simulink model "afe_dq_inv_psm"  (R2025a)
settings: Solver=ode1be  StartTime=0.0  StopTime=simlength  FixedStep=tc  MaxStep=tc
undefined symbols (not defined in the file): Adrso, Amplitude_U, Amplitude_V, Amplitude_W, b, Crso, CTRPIFF_CLIP_RELEASE, dead_time_AFE, dead_time_INV, deepNEGeta, deepNEGxi, deepPOSxi, emf_fb_p, emf_fb_p_ccaller_1, emf_fb_p_ccaller_2, emf_p, emf_p_ccaller_1, emf_p_ccaller_2, end_time_LVRT, fPWM_AFE, fPWM_INV, g0_500Hz, g1_500Hz, ibez, id_lim, Igrid_phase_normalization_factor, iq_lim, ixi_pos_ref_lim, Jm, kg, ki_afe, ki_i, ki_rc_grid, ki_vs, ki_w, kp_afe, kp_i, kp_rc_grid, kp_vs, kp_w, kw, Ld_norm, Ldrso, Lq_norm, Ls_norm, magnitude, motorc_m_scale, n1, n10, omega_bez, omega_grid_emulator_nom, omega_grid_nom, omega_m_bez, omega_m_sim, Phase_shift, pll_i1, pll_i1_ddsrt, pll_p, pll_p_ddsrt, pll_p_frt ... (+27)
libraries: fl_lib x114, nesl_utility x78, cstblocks x14, single_phase_transformer_lib x3, threephase_inductor_lib x2, simulink x2, flexshaft_lib x1, pmsm_uvw_with_harmonics_lib x1
(part 2 of 7)

== system afe_dq_inv_psm/grid/grid_emulator ==
  3ph_Dyg : Subsystem
  Controlled Voltage Source : fl_lib/Electrical/Electrical Sources/Controlled Voltage Source
  Controlled Voltage Source1 : fl_lib/Electrical/Electrical Sources/Controlled Voltage Source
  Controlled Voltage Source2 : fl_lib/Electrical/Electrical Sources/Controlled Voltage Source
  Electrical Reference : fl_lib/Electrical/Electrical Elements/Electrical Reference
  Simulink-PS Converter : nesl_utility/Simulink-PS Converter  PhysicalDomain=network_engine_domain  SubClassName=ps_input  LeftPortType=input  RightPortType=output  PseudoPeriodic=off  Frequencies=[]  NoiseDistribution=none  NoiseParameters=[]  Unit=V  AffineConversion=on  FilteringAndDerivatives=provide  SimscapeFilterOrder=1  InputFilterTimeConstant=0.001  UdotUserProvided=0
  Simulink-PS Converter1 : nesl_utility/Simulink-PS Converter  PhysicalDomain=network_engine_domain  SubClassName=ps_input  LeftPortType=input  RightPortType=output  PseudoPeriodic=off  Frequencies=[]  NoiseDistribution=none  NoiseParameters=[]  Unit=V  AffineConversion=on  FilteringAndDerivatives=provide  SimscapeFilterOrder=1  InputFilterTimeConstant=0.001  UdotUserProvided=0
  Simulink-PS Converter2 : nesl_utility/Simulink-PS Converter  PhysicalDomain=network_engine_domain  SubClassName=ps_input  LeftPortType=input  RightPortType=output  PseudoPeriodic=off  Frequencies=[]  NoiseDistribution=none  NoiseParameters=[]  Unit=V  AffineConversion=on  FilteringAndDerivatives=provide  SimscapeFilterOrder=1  InputFilterTimeConstant=0.001  UdotUserProvided=0
  Solver Configuration : nesl_utility/Solver Configuration  PhysicalDomain=network_engine_domain  SubClassName=solver  LeftPortType=input  RightPortType=generic  Tones=[]  Harmonics=[]  SimulateNoise=off  Profile=off  UseLocalSampling=off  EnableSwitchedLinearOptims=on  FrequencyDomain=off  UseCCode=off  RelTol=0.001  AbsTol=0.001  MinStep=1e-09  ToWorkspace=off  RevertToSquareIcSolve=off  NumHomotopyIterations=100  PhasorMode=off  PhasorModeNumHarmonics=1  ConsistencySolver=NEWTON_FTOL  IndexReductionMethod=DerivativeReplacement  DoDC=off  ResidualTolerance=1e-09  ConsistencyTolSource=GLOBAL  ConsistencyAbsTol=0.001  ConsistencyRelTol=0.001  ConsistencyTolFactor=0.001  UseLocalSolver=on  LocalSolverChoice=NE_BACKWARD_EULER_ADVANCER  ResolveIndetEquations=on  FunctionEvalNumThread=1  LocalSolverSampleTime=tc  DoFixedCost=on  MaxNonlinIter=3  MaxModeIter=2  ComputeImpulses=off  ImpulseIterations=2  LinearAlgebra=auto  LinearAlgebraNumThread=0  EquationFormulation=NE_TIME_EF  DelaysMemoryBudget=1024  AutomaticFiltering=on  FilteringTimeConstant=0.001  PartitionStorageMethod=AS_NEEDED  PartitionMemoryBudget=1024  PartitionMethod=ROBUST  MultibodyUseLocalSolver=off  MultibodyLocalSolverChoice=ODE1  MultibodyLocalSolverSampleTime=0.001
  grid_emulator : Subsystem
  threephase_vi_measures : Subsystem
  u1 : PMIOPort  Side=Right
  u2 : PMIOPort  Port=2  Side=Right
  u3 : PMIOPort  Port=3  Side=Right
  wires:
  grid_emulator/2(Vmb) -> Simulink-PS Converter1/1
  grid_emulator/3(Vmc) -> Simulink-PS Converter2/1
  grid_emulator/1(Vma) -> Simulink-PS Converter/1
  connections:
  Simulink-PS Converter/RConn1 -- Controlled Voltage Source/RConn1
  Simulink-PS Converter1/RConn1 -- Controlled Voltage Source1/RConn1
  Simulink-PS Converter2/RConn1 -- Controlled Voltage Source2/RConn1
  Electrical Reference/LConn1 -- Solver Configuration/RConn1 -- Controlled Voltage Source/RConn2 -- Controlled Voltage Source1/RConn2 -- Controlled Voltage Source2/RConn2
  3ph_Dyg/RConn1 -- u1/RConn1
  3ph_Dyg/RConn2 -- u2/RConn1
  3ph_Dyg/RConn3 -- u3/RConn1
  threephase_vi_measures/RConn1 -- 3ph_Dyg/LConn1
  threephase_vi_measures/RConn2 -- 3ph_Dyg/LConn2
  threephase_vi_measures/RConn3 -- 3ph_Dyg/LConn3
  Controlled Voltage Source/LConn1 -- threephase_vi_measures/LConn1
  Controlled Voltage Source1/LConn1 -- threephase_vi_measures/LConn2
  Controlled Voltage Source2/LConn1 -- threephase_vi_measures/LConn3

== system afe_dq_inv_psm/grid/instantaneus_power ==
  Vline : Inport
  Iline : Inport  Port=2
  Demux2 : Demux  Outputs=3
  Demux3 : Demux  Outputs=3
  Fcn1 : Fcn  Expr=u(1)/(sqrt(u(1)^2+u(2)^2))
  Gain2 : Gain  Gain=3/2
  Gain3 : Gain  Gain=3/2
  Mux1 : Mux  Inputs=2
  Product{,1..3} (4 alike) : Product  RndMeth=Zero
  Sum : Sum  Inputs=|++
  Sum1 : Sum  Inputs=|+-
  To Workspace1 : ToWorkspace  VariableName=va_line_rms_sim  SampleTime=ts_afe
      settings: MaxDataPoints=Ns_afe
  To Workspace2 : ToWorkspace  VariableName=vb_line_rms_sim  SampleTime=ts_afe
      settings: MaxDataPoints=Ns_afe
  To Workspace3 : ToWorkspace  VariableName=vc_line_rms_sim  SampleTime=ts_afe
      settings: MaxDataPoints=Ns_afe
  To Workspace4 : ToWorkspace  VariableName=ia_line_rms_sim  SampleTime=ts_afe
      settings: MaxDataPoints=Ns_afe
  To Workspace5 : ToWorkspace  VariableName=ib_line_rms_sim  SampleTime=ts_afe
      settings: MaxDataPoints=Ns_afe
  To Workspace6 : ToWorkspace  VariableName=ic_line_rms_sim  SampleTime=ts_afe
      settings: MaxDataPoints=Ns_afe
  To Workspace7 : ToWorkspace  VariableName=Pline_avg_sim  SampleTime=ts_afe
      settings: MaxDataPoints=Ns_afe
  To Workspace8 : ToWorkspace  VariableName=Qline_avg_sim  SampleTime=ts_afe
      settings: MaxDataPoints=Ns_afe
  abc2alphabeta : Subsystem
  "abc2alphabeta " : Subsystem
  mavg_11 : Subsystem
  mavg_12 : Subsystem
  rms : Subsystem
  rms1 : Subsystem
  rms2 : Subsystem
  rms3 : Subsystem
  rms4 : Subsystem
  rms5 : Subsystem
  tag scope: Pline_avg=global, Qline_avg=global, cos_phi_avg=global
  wires:
  Gain3/1 -> mavg_12/1(in), To Workspace8/1
  Gain2/1 -> mavg_11/1(in), To Workspace7/1
  Demux2/1 -> abc2alphabeta/1(a), rms/1(In1)
  Vline/1 -> Demux2/1
  Iline/1 -> Demux3/1
  abc2alphabeta/2(vline_beta) -> Product1/1, Product2/1
  "abc2alphabeta "/2(i_line_beta) -> Product3/1, Product1/2
  abc2alphabeta/1(vline_alpha) -> Product/1, Product3/2
  "abc2alphabeta "/1(i_line_alpha) -> Product2/2, Product/2
  Product/1 -> Sum/1
  Product1/1 -> Sum/2
  Product2/1 -> Sum1/1
  Product3/1 -> Sum1/2
  Sum1/1 -> Gain3/1
  Sum/1 -> Gain2/1
  Demux2/2 -> abc2alphabeta/2(b), rms1/1(In1)
  Demux2/3 -> abc2alphabeta/3(c), rms2/1(In1)
  Demux3/1 -> "abc2alphabeta "/1(a), rms3/1(In1)
  Demux3/2 -> "abc2alphabeta "/2(b), rms4/1(In1)
  Demux3/3 -> rms5/1(In1), "abc2alphabeta "/3(c)
  mavg_11/1(out) -> [Pline_avg]
  mavg_12/1(out) -> [Qline_avg]
  [Qline_avg] -> Mux1/2
  Mux1/1 -> Fcn1/1
  Fcn1/1 -> [cos_phi_avg]
  [Pline_avg] -> Mux1/1
  rms/1(Out1) -> To Workspace1/1
  rms2/1(Out1) -> To Workspace3/1
  rms1/1(Out1) -> To Workspace2/1
  rms5/1(Out1) -> To Workspace6/1
  rms4/1(Out1) -> To Workspace5/1
  rms3/1(Out1) -> To Workspace4/1

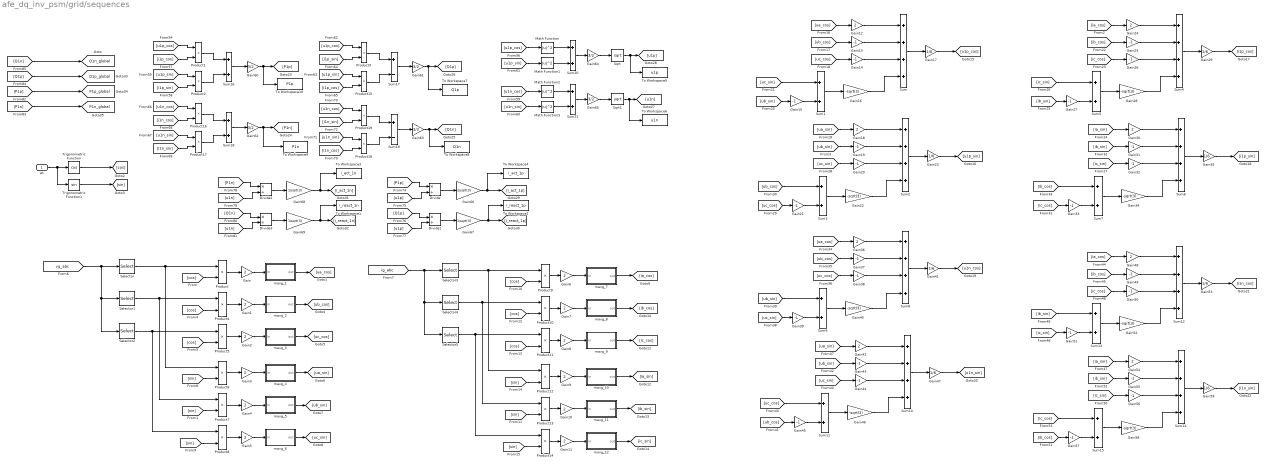
== system afe_dq_inv_psm/grid/sequences ==
  wt : Inport
  Divide{,1..3} (4 alike) : Product  Inputs=*/
  Gain{,1..12,18,24,30,36,42,48,54} (20 alike) : Gain  Gain=2
  Gain{13..15,19..21,25..27,31..33,37..39,43..45,49..51,55..57} (24 alike) : Gain  Gain=-1
  Gain{16,22,28,34,40,46,52,58} (8 alike) : Gain  Gain=-sqrt(3)
  Gain{17,23,29,35,41,47,53,59} (8 alike) : Gain  Gain=1/6
  Gain{60..65} (6 alike) : Gain  Gain=3/2
  Gain{66..69} (4 alike) : Gain  Gain=1/sqrt(3)
  Math Function{,1..3} (4 alike) : Math  Operator=magnitude^2  SignedPower=on
  Product{,1..19} (20 alike) : Product  RndMeth=Zero
  Selector : Selector  InputPortWidth=3  IndexOptions=Index vector (dialog)  Indices=1  OutputSizes=1
  Selector1 : Selector  InputPortWidth=3  IndexOptions=Index vector (dialog)  Indices=2  OutputSizes=1
  Selector2 : Selector  InputPortWidth=3  IndexOptions=Index vector (dialog)  Indices=3  OutputSizes=1
  Selector3 : Selector  InputPortWidth=3  IndexOptions=Index vector (dialog)  Indices=1  OutputSizes=1
  Selector4 : Selector  InputPortWidth=3  IndexOptions=Index vector (dialog)  Indices=2  OutputSizes=1
  Selector5 : Selector  InputPortWidth=3  IndexOptions=Index vector (dialog)  Indices=3  OutputSizes=1
  Sqrt : Sqrt
  Sqrt1 : Sqrt
  Sum{,2,4,6,8,10,12,14} (8 alike) : Sum  Inputs=++++
  Sum{1,3,5,7,9,11,13,15..16,18,20..21} (12 alike) : Sum
  Sum17 : Sum  Inputs=+-
  Sum19 : Sum  Inputs=+-
  To Workspace1 : ToWorkspace  VariableName=i_react_1n  SampleTime=ts_afe
      settings: MaxDataPoints=Ns_afe
  To Workspace10 : ToWorkspace  VariableName=P1p  SampleTime=ts_afe
      settings: MaxDataPoints=Ns_afe
  To Workspace2 : ToWorkspace  VariableName=i_react_1p  SampleTime=ts_afe
      settings: MaxDataPoints=Ns_afe
  To Workspace3 : ToWorkspace  VariableName=i_act_1n  SampleTime=ts_afe
      settings: MaxDataPoints=Ns_afe
  To Workspace4 : ToWorkspace  VariableName=i_act_1p  SampleTime=ts_afe
      settings: MaxDataPoints=Ns_afe
  To Workspace5 : ToWorkspace  VariableName=u1p  SampleTime=ts_afe
      settings: MaxDataPoints=Ns_afe
  To Workspace6 : ToWorkspace  VariableName=u1n  SampleTime=ts_afe
      settings: MaxDataPoints=Ns_afe
  To Workspace7 : ToWorkspace  VariableName=Q1p  SampleTime=ts_afe
      settings: MaxDataPoints=Ns_afe
  To Workspace8 : ToWorkspace  VariableName=Q1n  SampleTime=ts_afe
      settings: MaxDataPoints=Ns_afe
  To Workspace9 : ToWorkspace  VariableName=P1n  SampleTime=ts_afe
      settings: MaxDataPoints=Ns_afe
  Trigonometric Function : Trigonometry  Operator=cos
  Trigonometric Function1 : Trigonometry
  mavg_1 : Subsystem
  mavg_10 : Subsystem
  mavg_11 : Subsystem
  mavg_12 : Subsystem
  mavg_2 : Subsystem
  mavg_3 : Subsystem
  mavg_4 : Subsystem
  mavg_5 : Subsystem
  mavg_6 : Subsystem
  mavg_7 : Subsystem
  mavg_8 : Subsystem
  mavg_9 : Subsystem
  tag scope: P1n_global=global, P1p_global=global, Q1n_global=global, Q1p_global=global
  wires:
  [vg_abc] -> Selector2/1, Selector1/1, Selector/1
  Trigonometric Function1/1 -> [sin]
  Trigonometric Function/1 -> [cos]
  wt/1 -> Trigonometric Function/1, Trigonometric Function1/1
  [cos] -> Product/2
  Product/1 -> Gain/1
  [cos] -> Product4/2
  Product4/1 -> Gain1/1
  [cos] -> Product5/2
  Product5/1 -> Gain2/1
  [sin] -> Product6/2
  Selector/1 -> Product6/1, Product/1
  Product6/1 -> Gain3/1
  [sin] -> Product7/2
  Selector1/1 -> Product7/1, Product4/1
  Product7/1 -> Gain4/1
  [sin] -> Product8/2
  Selector2/1 -> Product8/1, Product5/1
  Product8/1 -> Gain5/1
  [ig_abc] -> Selector3/1, Selector4/1, Selector5/1
  [cos] -> Product9/2
  Product9/1 -> Gain6/1
  [cos] -> Product10/2
  Product10/1 -> Gain7/1
  [cos] -> Product11/2
  Product11/1 -> Gain8/1
  [sin] -> Product12/2
  Selector3/1 -> Product9/1, Product12/1
  Product12/1 -> Gain9/1
  [sin] -> Product13/2
  Selector4/1 -> Product10/1, Product13/1
  Product13/1 -> Gain10/1
  [sin] -> Product14/2
  Selector5/1 -> Product11/1, Product14/1
  Product14/1 -> Gain11/1
  Gain/1 -> mavg_1/1(in)
  mavg_1/1(out) -> [ua_cos]
  Gain1/1 -> mavg_2/1(in)
  Gain2/1 -> mavg_3/1(in)
  Gain3/1 -> mavg_4/1(in)
  Gain4/1 -> mavg_5/1(in)
  Gain5/1 -> mavg_6/1(in)
  Gain6/1 -> mavg_7/1(in)
  Gain7/1 -> mavg_8/1(in)
  Gain8/1 -> mavg_9/1(in)
  Gain9/1 -> mavg_10/1(in)
  Gain10/1 -> mavg_11/1(in)
  Gain11/1 -> mavg_12/1(in)
  [ua_cos] -> Gain12/1
  [ub_cos] -> Gain13/1
  [uc_cos] -> Gain14/1
  [uc_sin] -> Sum1/1
  Gain15/1 -> Sum1/2
  [ub_sin] -> Gain15/1
  Sum1/1 -> Gain16/1
  Gain16/1 -> Sum/4
  Gain14/1 -> Sum/3
  Gain13/1 -> Sum/2
  Gain12/1 -> Sum/1
  Sum/1 -> Gain17/1
  Gain17/1 -> [u1p_cos]
  [ua_sin] -> Gain18/1
  [ub_sin] -> Gain19/1
  [uc_sin] -> Gain20/1
  [ub_cos] -> Sum3/1
  Gain21/1 -> Sum3/2
  [uc_cos] -> Gain21/1
  Sum3/1 -> Gain22/1
  Gain22/1 -> Sum2/4
  Gain20/1 -> Sum2/3
  Gain19/1 -> Sum2/2
  Gain18/1 -> Sum2/1
  Sum2/1 -> Gain23/1
  Gain23/1 -> [u1p_sin]
  [ia_cos] -> Gain24/1
  [ib_cos] -> Gain25/1
  [ic_cos] -> Gain26/1
  [ic_sin] -> Sum5/1
  Gain27/1 -> Sum5/2
  [ib_sin] -> Gain27/1
  Sum5/1 -> Gain28/1
  Gain28/1 -> Sum4/4
  Gain26/1 -> Sum4/3
  Gain25/1 -> Sum4/2
  Gain24/1 -> Sum4/1
  Sum4/1 -> Gain29/1
  Gain29/1 -> [i1p_cos]
  [ia_sin] -> Gain30/1
  [ib_sin] -> Gain31/1
  [ic_sin] -> Gain32/1
  [ib_cos] -> Sum7/1
  Gain33/1 -> Sum7/2
  [ic_cos] -> Gain33/1
  Sum7/1 -> Gain34/1
  Gain34/1 -> Sum6/4
  Gain32/1 -> Sum6/3
  Gain31/1 -> Sum6/2
  Gain30/1 -> Sum6/1
  Sum6/1 -> Gain35/1
  Gain35/1 -> [i1p_sin]
  [ua_cos] -> Gain36/1
  [ub_cos] -> Gain37/1
  [uc_cos] -> Gain38/1
  [ub_sin] -> Sum9/1
  Gain39/1 -> Sum9/2
  [uc_sin] -> Gain39/1
  Sum9/1 -> Gain40/1
  Gain40/1 -> Sum8/4
  Gain38/1 -> Sum8/3
  Gain37/1 -> Sum8/2
  Gain36/1 -> Sum8/1
  Sum8/1 -> Gain41/1
  Gain41/1 -> [u1n_cos]
  [ua_sin] -> Gain42/1
  [ub_sin] -> Gain43/1
  [uc_sin] -> Gain44/1
  [uc_cos] -> Sum11/1
  Gain45/1 -> Sum11/2
  [ub_cos] -> Gain45/1
  Sum11/1 -> Gain46/1
  Gain46/1 -> Sum10/4
  Gain44/1 -> Sum10/3
  Gain43/1 -> Sum10/2
  Gain42/1 -> Sum10/1
  Sum10/1 -> Gain47/1
  Gain47/1 -> [u1n_sin]
  [ia_cos] -> Gain48/1
  [ib_cos] -> Gain49/1
  [ic_cos] -> Gain50/1
  [ib_sin] -> Sum13/1
  Gain51/1 -> Sum13/2
  [ic_sin] -> Gain51/1
  Sum13/1 -> Gain52/1
  Gain52/1 -> Sum12/4
  Gain50/1 -> Sum12/3
  Gain49/1 -> Sum12/2
  Gain48/1 -> Sum12/1
  Sum12/1 -> Gain53/1
  Gain53/1 -> [i1n_cos]
  [ia_sin] -> Gain54/1
  [ib_sin] -> Gain55/1
  [ic_sin] -> Gain56/1
  [ic_cos] -> Sum15/1
  Gain57/1 -> Sum15/2
  [ib_cos] -> Gain57/1
  Sum15/1 -> Gain58/1
  Gain58/1 -> Sum14/4
  Gain56/1 -> Sum14/3
  Gain55/1 -> Sum14/2
  Gain54/1 -> Sum14/1
  Sum14/1 -> Gain59/1
  Gain59/1 -> [i1n_sin]
  Sum16/1 -> Gain60/1
  Product1/1 -> Sum16/1
  Product2/1 -> Sum16/2
  Gain60/1 -> To Workspace10/1, [P1p]
  [u1p_cos] -> Product1/1
  [i1p_cos] -> Product1/2
  [u1p_sin] -> Product2/1
  [i1p_sin] -> Product2/2
  Sum17/1 -> Gain61/1
  Product3/1 -> Sum17/1
  Product15/1 -> Sum17/2
  Gain61/1 -> To Workspace7/1, [Q1p]
  [u1p_cos] -> Product3/1
  [i1p_sin] -> Product3/2
  [u1p_sin] -> Product15/1
  [i1p_cos] -> Product15/2
  Sum18/1 -> Gain62/1
  Product16/1 -> Sum18/1
  Product17/1 -> Sum18/2
  Gain62/1 -> To Workspace9/1, [P1n]
  [u1n_cos] -> Product16/1
  [i1n_cos] -> Product16/2
  [u1n_sin] -> Product17/1
  [i1n_sin] -> Product17/2
  Sum19/1 -> Gain63/1
  Product19/1 -> Sum19/1
  Product18/1 -> Sum19/2
  Gain63/1 -> To Workspace8/1, [Q1n]
  [u1n_cos] -> Product19/1
  [i1n_sin] -> Product19/2
  [u1n_sin] -> Product18/1
  [i1n_cos] -> Product18/2
  [u1p_cos] -> Math Function/1
  [u1p_sin] -> Math Function1/1
  Math Function/1 -> Sum20/1
  Math Function1/1 -> Sum20/2
  Sum20/1 -> Gain64/1
  Gain64/1 -> Sqrt/1
  Sqrt/1 -> To Workspace5/1, [u1p]
  [u1n_cos] -> Math Function2/1
  [u1n_sin] -> Math Function3/1
  Math Function2/1 -> Sum21/1
  Math Function3/1 -> Sum21/2
  Sum21/1 -> Gain65/1
  Gain65/1 -> Sqrt1/1
  Sqrt1/1 -> To Workspace6/1, [u1n]
  [P1p] -> Divide/1
  [u1p] -> Divide/2
  Divide/1 -> Gain66/1
  Gain66/1 -> To Workspace4/1, [i_act_1p]
  [Q1p] -> Divide1/1
  [u1p] -> Divide1/2
  Divide1/1 -> Gain67/1
  Gain67/1 -> To Workspace2/1, [i_react_1p]
  [P1n] -> Divide2/1
  [u1n] -> Divide2/2
  Divide2/1 -> Gain68/1
  Gain68/1 -> To Workspace3/1, [i_act_1n]
  [Q1n] -> Divide3/1
  [u1n] -> Divide3/2
  Divide3/1 -> Gain69/1
  Gain69/1 -> To Workspace1/1, [i_react_1n]
  mavg_2/1(out) -> [ub_cos]
  mavg_3/1(out) -> [uc_cos]
  mavg_4/1(out) -> [ua_sin]
  mavg_5/1(out) -> [ub_sin]
  mavg_6/1(out) -> [uc_sin]
  mavg_7/1(out) -> [ia_cos]
  mavg_8/1(out) -> [ib_cos]
  mavg_9/1(out) -> [ic_cos]
  mavg_10/1(out) -> [ia_sin]
  mavg_11/1(out) -> [ib_sin]
  mavg_12/1(out) -> [ic_sin]
  [Q1n] -> [Q1n_global]
  [Q1p] -> [Q1p_global]
  [P1p] -> [P1p_global]
  [P1n] -> [P1n_global]

== system afe_dq_inv_psm/grid/threephase_vi_measures ==
  Bus Creator : BusCreator  Inputs=6
  Current Sensor : fl_lib/Electrical/Electrical Sensors/Current Sensor
  Current Sensor1 : fl_lib/Electrical/Electrical Sensors/Current Sensor
  Current Sensor2 : fl_lib/Electrical/Electrical Sensors/Current Sensor
  Electrical Reference1 : fl_lib/Electrical/Electrical Elements/Electrical Reference
  Selector : Selector  InputPortWidth=6  IndexOptions=Index vector (dialog)  Indices=[1 2 3]  OutputSizes=1
  Selector1 : Selector  InputPortWidth=6  IndexOptions=Index vector (dialog)  Indices=[4 5 6]  OutputSizes=1
  Voltage Sensor : fl_lib/Electrical/Electrical Sensors/Voltage Sensor
  Voltage Sensor1 : fl_lib/Electrical/Electrical Sensors/Voltage Sensor
  Voltage Sensor2 : fl_lib/Electrical/Electrical Sensors/Voltage Sensor
  ia_grid : nesl_utility/PS-Simulink Converter  PhysicalDomain=network_engine_domain  SubClassName=ps_output  LeftPortType=input  RightPortType=output  PseudoPeriodic=off  Frequencies=[]  VectorFormat=1-D array  Unit=A  AffineConversion=off
  ib_grid : nesl_utility/PS-Simulink Converter  PhysicalDomain=network_engine_domain  SubClassName=ps_output  LeftPortType=input  RightPortType=output  PseudoPeriodic=off  Frequencies=[]  VectorFormat=1-D array  Unit=A  AffineConversion=off
  ic_grid : nesl_utility/PS-Simulink Converter  PhysicalDomain=network_engine_domain  SubClassName=ps_output  LeftPortType=input  RightPortType=output  PseudoPeriodic=off  Frequencies=[]  VectorFormat=1-D array  Unit=A  AffineConversion=off
  ig_abc/ug_abc : Scope  NumInputPorts=2
      settings: SampleTime=tc  ActiveDisplayYMinimum=-728.04682585664023  ActiveDisplayYMaximum=740.95420771528393  DataLoggingVariableName=ScopeData2
  power-meter : Scope  NumInputPorts=2
      settings: SampleTime=tc  ActiveDisplayYMinimum=-388201.13873747073  ActiveDisplayYMaximum=116083.0892842215  DataLoggingVariableName=ScopeData3
  ua_grid : nesl_utility/PS-Simulink Converter  PhysicalDomain=network_engine_domain  SubClassName=ps_output  LeftPortType=input  RightPortType=output  PseudoPeriodic=off  Frequencies=[]  VectorFormat=1-D array  Unit=V  AffineConversion=off
  ub_grid : nesl_utility/PS-Simulink Converter  PhysicalDomain=network_engine_domain  SubClassName=ps_output  LeftPortType=input  RightPortType=output  PseudoPeriodic=off  Frequencies=[]  VectorFormat=1-D array  Unit=V  AffineConversion=off
  uc_grid : nesl_utility/PS-Simulink Converter  PhysicalDomain=network_engine_domain  SubClassName=ps_output  LeftPortType=input  RightPortType=output  PseudoPeriodic=off  Frequencies=[]  VectorFormat=1-D array  Unit=V  AffineConversion=off
  Ua : PMIOPort  Side=Left
  ua : PMIOPort  Port=2  Side=Right
  Ub : PMIOPort  Port=3  Side=Left
  ub : PMIOPort  Port=4  Side=Right
  Uc : PMIOPort  Port=5  Side=Left
  uc : PMIOPort  Port=6  Side=Right
  tag scope: ig_abc=global, vg_abc=global
  wires:
  Bus Creator/1 -> Selector1/1, Selector/1  "vi_data"
  Selector/1 -> [vg_abc]
  ib_grid/1 -> Bus Creator/5  "ib"
  ia_grid/1 -> Bus Creator/4  "ia"
  ic_grid/1 -> Bus Creator/6  "ic"
  ua_grid/1 -> Bus Creator/1  "ua"
  ub_grid/1 -> Bus Creator/2  "ub"
  uc_grid/1 -> Bus Creator/3  "uc"
  Selector1/1 -> [ig_abc]
  [vg_abc] -> ig_abc/ug_abc/2
  [ig_abc] -> ig_abc/ug_abc/1
  [Pline_avg] -> power-meter/1
  [Qline_avg] -> power-meter/2
  connections:
  Current Sensor1/LConn1 -- Ub/RConn1 -- Voltage Sensor1/LConn1
  Electrical Reference1/LConn1 -- Voltage Sensor/RConn2 -- Voltage Sensor2/RConn2 -- Voltage Sensor1/RConn2
  Voltage Sensor/RConn1 -- ua_grid/LConn1
  Current Sensor/RConn2 -- ua/RConn1
  Voltage Sensor1/RConn1 -- ub_grid/LConn1
  Voltage Sensor2/LConn1 -- Current Sensor2/LConn1 -- Uc/RConn1
  Current Sensor/LConn1 -- Ua/RConn1 -- Voltage Sensor/LConn1
  Current Sensor1/RConn2 -- ub/RConn1
  Voltage Sensor2/RConn1 -- uc_grid/LConn1
  ib_grid/LConn1 -- Current Sensor1/RConn1
  ia_grid/LConn1 -- Current Sensor/RConn1
  ic_grid/LConn1 -- Current Sensor2/RConn1
  Current Sensor2/RConn2 -- uc/RConn1

== system afe_dq_inv_psm/motor_load_setting/flex-shaft ==
  flexible shaft : flexshaft_lib/flexible shaft  b1=1 N*m*s/rad  J1=1 kg*m^2  b2=1 N*m*s/rad  J2=1 kg*m^2  b_theta=1 N*m*s/rad  k_theta=1e4 N*m/rad  w_1_specify=off  w_1_priority=None  w_1=0 rad/s  w_1_nominal_specify=off  w_1_nominal_value=1  w_1_nominal_unit=rad/s  w_2_specify=off  w_2_priority=None  w_2=0 rad/s  w_2_nominal_specify=off  w_2_nominal_value=1  w_2_nominal_unit=rad/s  t_1_specify=off  t_1_priority=None  t_1=0 N*m  t_1_nominal_specify=off  t_1_nominal_value=1  t_1_nominal_unit=N*m  t_2_specify=off  t_2_priority=None  t_2=0 N*m  t_2_nominal_specify=off  t_2_nominal_value=1  t_2_nominal_unit=N*m  t_theta_specify=off  t_theta_priority=None  t_theta=0 N*m  t_theta_nominal_specify=off  t_theta_nominal_value=1  t_theta_nominal_unit=N*m
      settings: InternalSimscapePortConfiguration="{\"Bottom\":[],\"Left\":[{\"id\":\"S1\",\"label\":\"S1\",\"type\":\"foundation.mechanical.rotational.rotational\"}],\"Right\":[{\"id\":\"S2\",\"label\":\"S2\",\"type\":\"foundation.mechanical.rotational.rotational\"}],\"Top\":[]}"
  s2 : PMIOPort  Side=Right
  s1 : PMIOPort  Port=2  Side=Left
  connections:
  flexible shaft/RConn1 -- s2/RConn1
  flexible shaft/LConn1 -- s1/RConn1

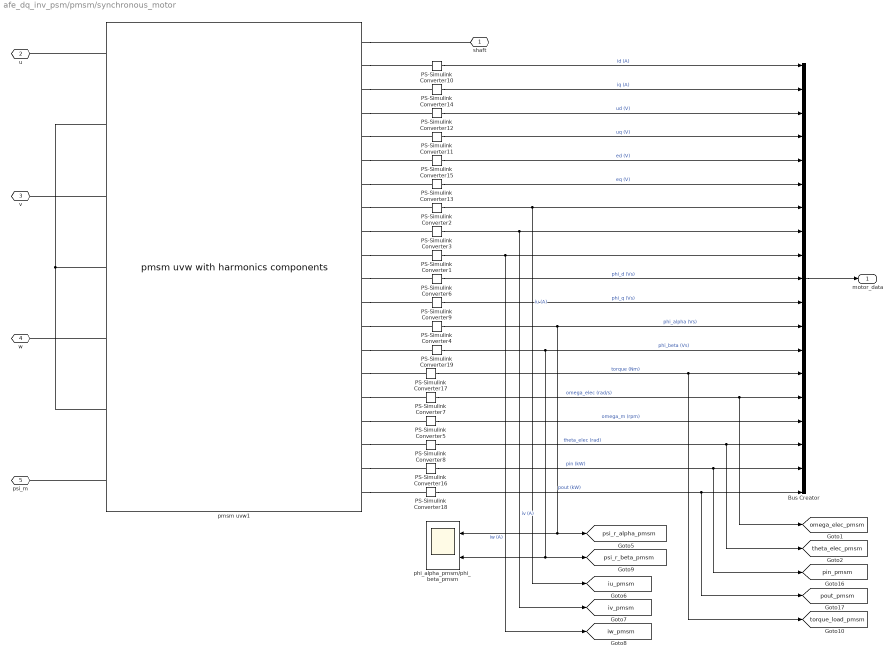
== system afe_dq_inv_psm/pmsm/synchronous_motor ==
  Bus Creator : BusCreator  Inputs=19
  PS-Simulink Converter{1..3,10,14} (5 alike) : nesl_utility/PS-Simulink Converter  PhysicalDomain=network_engine_domain  SubClassName=ps_output  LeftPortType=input  RightPortType=output  PseudoPeriodic=off  Frequencies=[]  VectorFormat=1-D array  Unit=A  AffineConversion=off
  PS-Simulink Converter{11..13,15} (4 alike) : nesl_utility/PS-Simulink Converter  PhysicalDomain=network_engine_domain  SubClassName=ps_output  LeftPortType=input  RightPortType=output  PseudoPeriodic=off  Frequencies=[]  VectorFormat=1-D array  Unit=V  AffineConversion=off
  PS-Simulink Converter16 : nesl_utility/PS-Simulink Converter  PhysicalDomain=network_engine_domain  SubClassName=ps_output  LeftPortType=input  RightPortType=output  PseudoPeriodic=off  Frequencies=[]  VectorFormat=1-D array  Unit=kW  AffineConversion=off
  PS-Simulink Converter17 : nesl_utility/PS-Simulink Converter  PhysicalDomain=network_engine_domain  SubClassName=ps_output  LeftPortType=input  RightPortType=output  PseudoPeriodic=off  Frequencies=[]  VectorFormat=1-D array  Unit=N*m  AffineConversion=off
  PS-Simulink Converter18 : nesl_utility/PS-Simulink Converter  PhysicalDomain=network_engine_domain  SubClassName=ps_output  LeftPortType=input  RightPortType=output  PseudoPeriodic=off  Frequencies=[]  VectorFormat=1-D array  Unit=kW  AffineConversion=off
  PS-Simulink Converter{4,6,9,19} (4 alike) : nesl_utility/PS-Simulink Converter  PhysicalDomain=network_engine_domain  SubClassName=ps_output  LeftPortType=input  RightPortType=output  PseudoPeriodic=off  Frequencies=[]  VectorFormat=1-D array  Unit=V*s  AffineConversion=off
  PS-Simulink Converter5 : nesl_utility/PS-Simulink Converter  PhysicalDomain=network_engine_domain  SubClassName=ps_output  LeftPortType=input  RightPortType=output  PseudoPeriodic=off  Frequencies=[]  VectorFormat=1-D array  Unit=rpm  AffineConversion=off
  PS-Simulink Converter7 : nesl_utility/PS-Simulink Converter  PhysicalDomain=network_engine_domain  SubClassName=ps_output  LeftPortType=input  RightPortType=output  PseudoPeriodic=off  Frequencies=[]  VectorFormat=1-D array  Unit=rad/s  AffineConversion=off
  PS-Simulink Converter8 : nesl_utility/PS-Simulink Converter  PhysicalDomain=network_engine_domain  SubClassName=ps_output  LeftPortType=input  RightPortType=output  PseudoPeriodic=off  Frequencies=[]  VectorFormat=1-D array  Unit=rad  AffineConversion=off
  phi_alpha_pmsm/phi_beta_pmsm : Scope  NumInputPorts=2
      settings: SampleTime=tc  ActiveDisplayYMinimum=-4.80078  ActiveDisplayYMaximum=4.80088  DataLoggingVariableName=ScopeData2
  pmsm uvw1 : pmsm_uvw_with_harmonics_lib/pmsm uvw with harmonics components  number_poles=number_poles  psi_m_p=psi_m V*s  Lmu=Lmu H  La=La H  Lb=Lb H  Rs=Rs Ohm  J=Jm kg*m^2  b=b N*m*s/rad  b_square=0 %b_square N*m*s^2/rad^2  h5=4 percent  h7=1 percent  angle_error=0 rad  omega_specify=off  omega_priority=None  omega=0 rad/s  omega_nominal_specify=off  omega_nominal_unit=rad/s  omega_nominal_value=1  theta_specify=off  theta_priority=High  theta=0 rad  theta_nominal_specify=off  theta_nominal_unit=rad  theta_nominal_value=1  iu_specify=off  iu_priority=None  iu=0 A  iu_nominal_specify=off  iu_nominal_unit=A  iu_nominal_value=1  iv_specify=off  iv_priority=None  iv=0 A  iv_nominal_specify=off  iv_nominal_unit=A  iv_nominal_value=1  iw_specify=off  iw_priority=None  iw=0 A  iw_nominal_specify=off  iw_nominal_unit=A  iw_nominal_value=1  id_specify=off  id_priority=None  id=0 A  id_nominal_specify=off  id_nominal_unit=A  id_nominal_value=1  iq_specify=off  iq_priority=None  iq=0 A  iq_nominal_specify=off  iq_nominal_unit=A  iq_nominal_value=1  uv_specify=off  uv_priority=None  uv=0 V  uv_nominal_specify=off  uv_nominal_unit=V  uv_nominal_value=1  uu_specify=off  uu_priority=None  uu=0 V  uu_nominal_specify=off  uu_nominal_unit=V  uu_nominal_value=1  uw_specify=off  uw_priority=None  uw=0 V  uw_nominal_specify=off  uw_nominal_unit=V  uw_nominal_value=1  ud_specify=off  ud_priority=None  ud=0 V  ud_nominal_specify=off  ud_nominal_unit=V  ud_nominal_value=1  uq_specify=off  uq_priority=None  uq=0 V  uq_nominal_specify=off  uq_nominal_unit=V  uq_nominal_value=1  psi_r_u_specify=on  psi_r_u_priority=High  psi_r_u=psi_m V*s  psi_r_u_nominal_specify=off  psi_r_u_nominal_unit=V*s  psi_r_u_nominal_value=1  psi_r_v_specify=on  psi_r_v_priority=High  psi_r_v=-psi_m/2 V*s  psi_r_v_nominal_specify=off  psi_r_v_nominal_unit=V*s  psi_r_v_nominal_value=1  psi_r_w_specify=on  psi_r_w_priority=High  psi_r_w=-psi_m/2 V*s  psi_r_w_nominal_specify=off  psi_r_w_nominal_unit=V*s  psi_r_w_nominal_value=1  psi_s_d_specify=off  psi_s_d_priority=None  psi_s_d=0.0 V*s  psi_s_d_nominal_specify=off  psi_s_d_nominal_unit=V*s  psi_s_d_nominal_value=1  psi_s_q_specify=off  psi_s_q_priority=None  psi_s_q=0.0 V*s  psi_s_q_nominal_specify=off  psi_s_q_nominal_unit=V*s  psi_s_q_nominal_value=1  psi_r_d_specify=off  psi_r_d_priority=High  psi_r_d=phi_m V*s  psi_r_d_nominal_specify=off  psi_r_d_nominal_unit=V*s  psi_r_d_nominal_value=1  psi_r_q_specify=off  psi_r_q_priority=High  psi_r_q=0.0 V*s  psi_r_q_nominal_specify=off  psi_r_q_nominal_unit=V*s  psi_r_q_nominal_value=1  psi_r_alpha_specify=off  psi_r_alpha_priority=High  psi_r_alpha=psi_m V*s  psi_r_alpha_nominal_specify=off  psi_r_alpha_nominal_unit=V*s  psi_r_alpha_nominal_value=1  psi_r_beta_specify=off  psi_r_beta_priority=High  psi_r_beta=0 V*s  psi_r_beta_nominal_specify=off  psi_r_beta_nominal_unit=V*s  psi_r_beta_nominal_value=1  psi_s_alpha_specify=off  psi_s_alpha_priority=None  psi_s_alpha=0.0 V*s  psi_s_alpha_nominal_specify=off  psi_s_alpha_nominal_unit=V*s  psi_s_alpha_nominal_value=1  psi_s_beta_specify=off  psi_s_beta_priority=None  psi_s_beta=0.0 V*s  psi_s_beta_nominal_specify=off  psi_s_beta_nominal_unit=V*s  psi_s_beta_nominal_value=1  tau_l_specify=off  tau_l_priority=None  tau_l=0 N*m  tau_l_nominal_specify=off  tau_l_nominal_unit=N*m  tau_l_nominal_value=1  tau_m_specify=off  tau_m_priority=None  tau_m=0 N*m  tau_m_nominal_specify=off  tau_m_nominal_unit=N*m  tau_m_nominal_value=1
      settings: InternalSimscapePortConfiguration="{\"Bottom\":[],\"Left\":[{\"id\":\"uu_p\",\"label\":\"_uu+_\",\"type\":\"foundation.electrical.electrical\"},{\"id\":\"uu_n\",\"label\":\"_uu-_\",\"type\":\"foundation.electrical.electrical\"},{\"id\":\"uv_p\",\"label\":\"_uv+_\",\"type\":\"foundation.electrical.electrical\"},{\"id\":\"uv_n\",\"label\":\"_uv-_\",\"type\":\"foundation.electrical.electrical\"},{\"id\":\"uw_p\",\"label\":\"_uw+_\",\"type\":\"foundation.electrical.electrical\"},{\"id\":\"uw_n\",\"label\":\"_uw-_\",\"type\":\"foundation.electrical.electrical\"},{\"id\":\"psi_m\",\"label\":\"_psi_m_\",\"type\":\"input\"}],\"Right\":[{\"id\":\"S\",\"label\":\"_S_\",\"type\":\"foundation.mechanical.rotational.rotational\"},{\"id\":\"id_out\",\"label\":\"_id_\",\"type\":\"output\"},{\"id\":\"iq_out\",\"label\":\"_iq_\",\"type\":\"output\"},{\"id\":\"ud_out\",\"label\":\"_ud_\",\"type\":\"output\"},{\"id\":\"uq_out\",\"label\":\"_uq_\",\"type\":\"output\"},{\"id\":\"ed_out\",\"label\":\"_ed_\",\"type\":\"output\"},{\"id\":\"eq_out\",\"label\":\"_eq_\",\"type\":\"output\"},{\"id\":\"iu_out\",\"label\":\"_iu_\",\"type\":\"output\"},{\"id\":\"iv_out\",\"label\":\"_iv_\",\"type\":\"output\"},{\"id\":\"iw_out\",\"label\":\"_iw_\",\"type\":\"output\"},{\"id\":\"psi_r_d_out\",\"label\":\"_psi_r_d_\",\"type\":\"output\"},{\"id\":\"psi_r_q_out\",\"label\":\"_psi_r_q\",\"type\":\"output\"},{\"id\":\"psi_r_alpha_out\",\"label\":\"_psi_r_alpha_\",\"type\":\"output\"},{\"id\":\"psi_r_beta_out\",\"label\":\"_psi_r_beta\",\"type\":\"output\"},{\"id\":\"tau_out\",\"label\":\"_torque_\",\"type\":\"output\"},{\"id\":\"omega_out\",\"label\":\"_omega_elec_\",\"type\":\"output\"},{\"id\":\"omega_m_out\",\"label\":\"_omega_m_\",\"type\":\"output\"},{\"id\":\"theta_out\",\"label\":\"_theta_elec_\",\"type\":\"output\"},{\"id\":\"pin_out\",\"label\":\"_pin_\",\"type\":\"output\"},{\"id\":\"pout_out\",\"label\":\"_pout_\",\"type\":\"output\"}],\"Top\":[]}"
  shaft : PMIOPort  Side=Right
  u : PMIOPort  Port=2  Side=Left
  v : PMIOPort  Port=3  Side=Left
  w : PMIOPort  Port=4  Side=Left
  psi_m : PMIOPort  Port=5  Side=Left
  motor_data : Outport
  tag scope: iu_pmsm=global, iv_pmsm=global, iw_pmsm=global, omega_elec_pmsm=global, pin_pmsm=global, pout_pmsm=global, psi_r_alpha_pmsm=global, psi_r_beta_pmsm=global, theta_elec_pmsm=global, torque_load_pmsm=global
  wires:
  PS-Simulink Converter10/1 -> Bus Creator/1  "id (A)"
  PS-Simulink Converter14/1 -> Bus Creator/2  "iq (A)"
  PS-Simulink Converter12/1 -> Bus Creator/3  "ud (V)"
  PS-Simulink Converter11/1 -> Bus Creator/4  "uq (V)"
  PS-Simulink Converter15/1 -> Bus Creator/5  "ed (V)"
  PS-Simulink Converter13/1 -> Bus Creator/6  "eq (V)"
  PS-Simulink Converter2/1 -> Bus Creator/7, [iu_pmsm]  "iu (A)"
  PS-Simulink Converter3/1 -> Bus Creator/8, [iv_pmsm]  "iv (A)"
  PS-Simulink Converter1/1 -> Bus Creator/9, [iw_pmsm]  "iw (A)"
  PS-Simulink Converter6/1 -> Bus Creator/10  "phi_d (Vs)"
  PS-Simulink Converter9/1 -> Bus Creator/11  "phi_q (Vs)"
  Bus Creator/1 -> motor_data/1
  PS-Simulink Converter18/1 -> Bus Creator/19, [pout_pmsm]  "pout (kW)"
  PS-Simulink Converter16/1 -> Bus Creator/18, [pin_pmsm]  "pin (kW)"
  PS-Simulink Converter8/1 -> Bus Creator/17, [theta_elec_pmsm]  "theta_elec (rad)"
  PS-Simulink Converter5/1 -> Bus Creator/16  "omega_m (rpm)"
  PS-Simulink Converter7/1 -> Bus Creator/15, [omega_elec_pmsm]  "omega_elec (rad/s)"
  PS-Simulink Converter17/1 -> [torque_load_pmsm], Bus Creator/14  "torque (Nm)"
  PS-Simulink Converter4/1 -> Bus Creator/12, phi_alpha_pmsm/phi_beta_pmsm/1, [psi_r_alpha_pmsm]  "phi_alpha (Vs)"
  PS-Simulink Converter19/1 -> Bus Creator/13, [psi_r_beta_pmsm], phi_alpha_pmsm/phi_beta_pmsm/2  "phi_beta (Vs)"
  connections:
  pmsm uvw1/RConn8 -- PS-Simulink Converter2/LConn1
  pmsm uvw1/RConn9 -- PS-Simulink Converter3/LConn1
  pmsm uvw1/RConn3 -- PS-Simulink Converter14/LConn1
  pmsm uvw1/RConn4 -- PS-Simulink Converter12/LConn1
  pmsm uvw1/RConn2 -- PS-Simulink Converter10/LConn1
  pmsm uvw1/LConn4 -- pmsm uvw1/LConn2 -- pmsm uvw1/LConn6
  pmsm uvw1/RConn7 -- PS-Simulink Converter13/LConn1
  pmsm uvw1/LConn1 -- u/RConn1
  pmsm uvw1/RConn12 -- PS-Simulink Converter9/LConn1
  pmsm uvw1/RConn10 -- PS-Simulink Converter1/LConn1
  pmsm uvw1/LConn5 -- w/RConn1
  pmsm uvw1/LConn7 -- psi_m/RConn1
  pmsm uvw1/RConn5 -- PS-Simulink Converter11/LConn1
  pmsm uvw1/RConn11 -- PS-Simulink Converter6/LConn1
  pmsm uvw1/RConn6 -- PS-Simulink Converter15/LConn1
  pmsm uvw1/LConn3 -- v/RConn1
  pmsm uvw1/RConn1 -- shaft/RConn1
  pmsm uvw1/RConn15 -- PS-Simulink Converter17/LConn1
  pmsm uvw1/RConn16 -- PS-Simulink Converter7/LConn1
  pmsm uvw1/RConn17 -- PS-Simulink Converter5/LConn1
  pmsm uvw1/RConn18 -- PS-Simulink Converter8/LConn1
  pmsm uvw1/RConn19 -- PS-Simulink Converter16/LConn1
  pmsm uvw1/RConn20 -- PS-Simulink Converter18/LConn1
  pmsm uvw1/RConn13 -- PS-Simulink Converter4/LConn1
  pmsm uvw1/RConn14 -- PS-Simulink Converter19/LConn1

== system afe_dq_inv_psm/afe_dq_inv_psm_mod1/LCL_filter/threephase_vi_measures_stack ==
  Bus Creator : BusCreator  Inputs=6
  Current Sensor : fl_lib/Electrical/Electrical Sensors/Current Sensor
  Current Sensor1 : fl_lib/Electrical/Electrical Sensors/Current Sensor
  Current Sensor2 : fl_lib/Electrical/Electrical Sensors/Current Sensor
  Electrical Reference1 : fl_lib/Electrical/Electrical Elements/Electrical Reference
  Selector : Selector  InputPortWidth=6  IndexOptions=Index vector (dialog)  Indices=[1 2 3]  OutputSizes=1
  Selector1 : Selector  InputPortWidth=6  IndexOptions=Index vector (dialog)  Indices=[4 5 6]  OutputSizes=1
  Voltage Sensor : fl_lib/Electrical/Electrical Sensors/Voltage Sensor
  Voltage Sensor1 : fl_lib/Electrical/Electrical Sensors/Voltage Sensor
  Voltage Sensor2 : fl_lib/Electrical/Electrical Sensors/Voltage Sensor
  ia_afe : nesl_utility/PS-Simulink Converter  PhysicalDomain=network_engine_domain  SubClassName=ps_output  LeftPortType=input  RightPortType=output  PseudoPeriodic=off  Frequencies=[]  VectorFormat=1-D array  Unit=A  AffineConversion=off
  ib_afe : nesl_utility/PS-Simulink Converter  PhysicalDomain=network_engine_domain  SubClassName=ps_output  LeftPortType=input  RightPortType=output  PseudoPeriodic=off  Frequencies=[]  VectorFormat=1-D array  Unit=A  AffineConversion=off
  ic_afe : nesl_utility/PS-Simulink Converter  PhysicalDomain=network_engine_domain  SubClassName=ps_output  LeftPortType=input  RightPortType=output  PseudoPeriodic=off  Frequencies=[]  VectorFormat=1-D array  Unit=A  AffineConversion=off
  is_abc/us_abc : Scope  NumInputPorts=2
      settings: SampleTime=tc  ActiveDisplayYMinimum=-1012.5759955513984  ActiveDisplayYMaximum=1081.7928142523619
  ua_afe : nesl_utility/PS-Simulink Converter  PhysicalDomain=network_engine_domain  SubClassName=ps_output  LeftPortType=input  RightPortType=output  PseudoPeriodic=off  Frequencies=[]  VectorFormat=1-D array  Unit=V  AffineConversion=off
  ub_afe : nesl_utility/PS-Simulink Converter  PhysicalDomain=network_engine_domain  SubClassName=ps_output  LeftPortType=input  RightPortType=output  PseudoPeriodic=off  Frequencies=[]  VectorFormat=1-D array  Unit=V  AffineConversion=off
  uc_afe : nesl_utility/PS-Simulink Converter  PhysicalDomain=network_engine_domain  SubClassName=ps_output  LeftPortType=input  RightPortType=output  PseudoPeriodic=off  Frequencies=[]  VectorFormat=1-D array  Unit=V  AffineConversion=off
  Ua : PMIOPort  Side=Left
  ua : PMIOPort  Port=2  Side=Right
  Ub : PMIOPort  Port=3  Side=Left
  ub : PMIOPort  Port=4  Side=Right
  Uc : PMIOPort  Port=5  Side=Left
  uc : PMIOPort  Port=6  Side=Right
  tag scope: is_abc=global, vs_abc=global
  wires:
  Bus Creator/1 -> Selector1/1, Selector/1  "vi_data"
  Selector/1 -> [vs_abc]
  ib_afe/1 -> Bus Creator/5  "ib_afe"
  ia_afe/1 -> Bus Creator/4  "ia_afe"
  ic_afe/1 -> Bus Creator/6  "ic_afe"
  ua_afe/1 -> Bus Creator/1  "ua_afe"
  ub_afe/1 -> Bus Creator/2  "ub_afe"
  uc_afe/1 -> Bus Creator/3  "uc_afe"
  Selector1/1 -> [is_abc]
  [is_abc] -> is_abc/us_abc/1  "is_abc"
  [vs_abc] -> is_abc/us_abc/2  "us_abc"
  connections:
  Current Sensor1/LConn1 -- Ub/RConn1 -- Voltage Sensor1/LConn1
  Electrical Reference1/LConn1 -- Voltage Sensor/RConn2 -- Voltage Sensor2/RConn2 -- Voltage Sensor1/RConn2
  Voltage Sensor/RConn1 -- ua_afe/LConn1
  Current Sensor/RConn2 -- ua/RConn1
  Voltage Sensor1/RConn1 -- ub_afe/LConn1
  Voltage Sensor2/LConn1 -- Uc/RConn1 -- Current Sensor2/LConn1
  Current Sensor/LConn1 -- Ua/RConn1 -- Voltage Sensor/LConn1
  Current Sensor1/RConn2 -- ub/RConn1
  Voltage Sensor2/RConn1 -- uc_afe/LConn1
  ib_afe/LConn1 -- Current Sensor1/RConn1
  ia_afe/LConn1 -- Current Sensor/RConn1
  ic_afe/LConn1 -- Current Sensor2/RConn1
  Current Sensor2/RConn2 -- uc/RConn1

== system afe_dq_inv_psm/afe_dq_inv_psm_mod1/L_filter/threephase_vi_measures_stack ==
  Bus Creator : BusCreator  Inputs=6
  Current Sensor : fl_lib/Electrical/Electrical Sensors/Current Sensor
  Current Sensor1 : fl_lib/Electrical/Electrical Sensors/Current Sensor
  Current Sensor2 : fl_lib/Electrical/Electrical Sensors/Current Sensor
  Electrical Reference1 : fl_lib/Electrical/Electrical Elements/Electrical Reference
  Selector : Selector  InputPortWidth=6  IndexOptions=Index vector (dialog)  Indices=[1 2 3]  OutputSizes=1
  Selector1 : Selector  InputPortWidth=6  IndexOptions=Index vector (dialog)  Indices=[4 5 6]  OutputSizes=1
  Voltage Sensor : fl_lib/Electrical/Electrical Sensors/Voltage Sensor
  Voltage Sensor1 : fl_lib/Electrical/Electrical Sensors/Voltage Sensor
  Voltage Sensor2 : fl_lib/Electrical/Electrical Sensors/Voltage Sensor
  is_uvw/us_uvw : Scope  NumInputPorts=2
      settings: SampleTime=tc  ActiveDisplayYMinimum=-1039.48512380396  ActiveDisplayYMaximum=979.57633627999246
  iu_inv : nesl_utility/PS-Simulink Converter  PhysicalDomain=network_engine_domain  SubClassName=ps_output  LeftPortType=input  RightPortType=output  PseudoPeriodic=off  Frequencies=[]  VectorFormat=1-D array  Unit=A  AffineConversion=off
  iv_inv : nesl_utility/PS-Simulink Converter  PhysicalDomain=network_engine_domain  SubClassName=ps_output  LeftPortType=input  RightPortType=output  PseudoPeriodic=off  Frequencies=[]  VectorFormat=1-D array  Unit=A  AffineConversion=off
  iw_inv : nesl_utility/PS-Simulink Converter  PhysicalDomain=network_engine_domain  SubClassName=ps_output  LeftPortType=input  RightPortType=output  PseudoPeriodic=off  Frequencies=[]  VectorFormat=1-D array  Unit=A  AffineConversion=off
  uu_afe : nesl_utility/PS-Simulink Converter  PhysicalDomain=network_engine_domain  SubClassName=ps_output  LeftPortType=input  RightPortType=output  PseudoPeriodic=off  Frequencies=[]  VectorFormat=1-D array  Unit=V  AffineConversion=off
  uv_afe : nesl_utility/PS-Simulink Converter  PhysicalDomain=network_engine_domain  SubClassName=ps_output  LeftPortType=input  RightPortType=output  PseudoPeriodic=off  Frequencies=[]  VectorFormat=1-D array  Unit=V  AffineConversion=off
  uw_afe : nesl_utility/PS-Simulink Converter  PhysicalDomain=network_engine_domain  SubClassName=ps_output  LeftPortType=input  RightPortType=output  PseudoPeriodic=off  Frequencies=[]  VectorFormat=1-D array  Unit=V  AffineConversion=off
  Uu : PMIOPort  Side=Left
  uu : PMIOPort  Port=2  Side=Right
  Uv : PMIOPort  Port=3  Side=Left
  uv : PMIOPort  Port=4  Side=Right
  Uw : PMIOPort  Port=5  Side=Left
  uw : PMIOPort  Port=6  Side=Right
  tag scope: is_uvw=global, vs_uvw=global
  wires:
  Bus Creator/1 -> Selector1/1, Selector/1  "vi_data"
  Selector/1 -> [vs_uvw]
  iv_inv/1 -> Bus Creator/5  "iv_inv"
  iu_inv/1 -> Bus Creator/4  "iu_inv"
  iw_inv/1 -> Bus Creator/6  "iw_inv"
  uu_afe/1 -> Bus Creator/1  "uu_afe"
  uv_afe/1 -> Bus Creator/2  "uv_afe"
  uw_afe/1 -> Bus Creator/3  "uw_afe"
  Selector1/1 -> [is_uvw]
  [is_uvw] -> is_uvw/us_uvw/1
  [vs_uvw] -> is_uvw/us_uvw/2
  connections:
  Current Sensor1/LConn1 -- Uv/RConn1 -- Voltage Sensor1/LConn1
  Electrical Reference1/LConn1 -- Voltage Sensor/RConn2 -- Voltage Sensor2/RConn2 -- Voltage Sensor1/RConn2
  Voltage Sensor/RConn1 -- uu_afe/LConn1
  Current Sensor/RConn2 -- uu/RConn1
  Voltage Sensor1/RConn1 -- uv_afe/LConn1
  Voltage Sensor2/LConn1 -- Uw/RConn1 -- Current Sensor2/LConn1
  Current Sensor/LConn1 -- Uu/RConn1 -- Voltage Sensor/LConn1
  Current Sensor1/RConn2 -- uv/RConn1
  Voltage Sensor2/RConn1 -- uw_afe/LConn1
  iv_inv/LConn1 -- Current Sensor1/RConn1
  iu_inv/LConn1 -- Current Sensor/RConn1
  iw_inv/LConn1 -- Current Sensor2/RConn1
  Current Sensor2/RConn2 -- uw/RConn1

== system afe_dq_inv_psm/afe_dq_inv_psm_mod1/afe/dclink_measure ==
  Controlled Voltage Source : fl_lib/Electrical/Electrical Sources/Controlled Voltage Source
  Current Sensor1 : fl_lib/Electrical/Electrical Sensors/Current Sensor
  Electrical Reference : fl_lib/Electrical/Electrical Elements/Electrical Reference
  Gain : Gain  Gain=107.4e3
  Gain1 : Gain  Gain=1/Vdc_bez
  Quantizer : Quantizer  QuantizationInterval=VoltageQuantization
  R_derating : Subsystem  Commented=on
  Resistor : fl_lib/Electrical/Electrical Elements/Resistor  R=107.4 kOhm  i_specify=off  i_priority=None  i=0 A  i_nominal_specify=off  i_nominal_value=1  i_nominal_unit=A  v_specify=off  v_priority=None  v=0 V  v_nominal_specify=off  v_nominal_value=1  v_nominal_unit=V
  Saturation : Saturate  UpperLimit=inf  LowerLimit=1
  Simulink-PS Converter : nesl_utility/Simulink-PS Converter  PhysicalDomain=network_engine_domain  SubClassName=ps_input  LeftPortType=input  RightPortType=output  PseudoPeriodic=off  Frequencies=[]  NoiseDistribution=none  NoiseParameters=[]  Unit=Ohm  AffineConversion=off  FilteringAndDerivatives=provide  SimscapeFilterOrder=1  InputFilterTimeConstant=0.001  UdotUserProvided=0
  Variable Resistor : fl_lib/Electrical/Electrical Elements/Variable Resistor  Rmin=0 Ohm  thermalEnable=false  thermal_mass=1 J/K  i_specify=off  i_priority=None  i=0 A  i_nominal_specify=off  i_nominal_value=1  i_nominal_unit=A  v_specify=off  v_priority=None  v=0 V  v_nominal_specify=off  v_nominal_value=1  v_nominal_unit=V  T_specify=off  T_priority=None  T=300 K  T_nominal_specify=off  T_nominal_value=1  T_nominal_unit=K
  dclink_voltage_measure_comparison : Scope  NumInputPorts=3
      settings: SampleTime=tc  ActiveDisplayYMinimum=-105.37024381606814  ActiveDisplayYMaximum=1410.5586556062556
  im_udc : nesl_utility/PS-Simulink Converter  PhysicalDomain=network_engine_domain  SubClassName=ps_output  LeftPortType=input  RightPortType=output  PseudoPeriodic=off  Frequencies=[]  VectorFormat=1-D array  Unit=A  AffineConversion=on
  udc : PMIOPort  Side=Left
  tag scope: vdc_pu=global
  wires:
  Gain/1 -> Saturation/1, dclink_voltage_measure_comparison/1  "measure_si"
  Quantizer/1 -> Gain1/1
  Saturation/1 -> Quantizer/1
  im_udc/1 -> Gain/1
  Gain1/1 -> dclink_voltage_measure_comparison/2, [vdc_pu]  "measure_pu"
  [udc] -> dclink_voltage_measure_comparison/3  "real"
  R_derating/1(DR) -> Simulink-PS Converter/1
  connections:
  udc/RConn1 -- Controlled Voltage Source/RConn1
  Resistor/RConn1 -- Variable Resistor/LConn2
  Current Sensor1/RConn1 -- im_udc/LConn1
  Current Sensor1/RConn2 -- Electrical Reference/LConn1 -- Controlled Voltage Source/RConn2
  Current Sensor1/LConn1 -- Variable Resistor/RConn1
  Simulink-PS Converter/RConn1 -- Variable Resistor/LConn1
  Controlled Voltage Source/LConn1 -- Resistor/LConn1

== system afe_dq_inv_psm/afe_dq_inv_psm_mod1/afe/sv_pwm ==
  ab : Inport
  enable : Inport  Port=2
  Bus Selector : BusSelector  OutputSignals=da,db,dc
  Bus Selector1 : BusSelector  OutputSignals=ualpha_afe,ubeta_afe
  C Caller : CCaller  FunctionName=sv_pwm_process_simulink  PortSpecificationStruct="%)30     .    V @   8    (     @         %    \"     4    !     0         %  0 \"0    $    _    07)G3F%M90  4&]R=$YA;64 4V-O<&4     26YD97@     5'EP90      4VEZ90      27-';&]B86P   X    P    !@    @    $          4    (     0    ,    !         !   P!O=70 #@   #     &    \"     0         !0    @    !     P    $         $  # &]U=  .    .     8    (    !          %    \"     $    &     0         0   ...(+2669 chars)"  SampleTime=ts_afe
  Constant : Constant  Value=ts_afe
  Data Type Conversion1 : DataTypeConversion  OutDataTypeStr=double  SaturateOnIntegerOverflow=off  RndMeth=Floor
  Data Type Conversion15 : DataTypeConversion  OutDataTypeStr=single  SaturateOnIntegerOverflow=off  RndMeth=Floor
  Data Type Conversion16 : DataTypeConversion  OutDataTypeStr=single  SaturateOnIntegerOverflow=off  RndMeth=Floor
  Data Type Conversion17 : DataTypeConversion  OutDataTypeStr=uint32  SaturateOnIntegerOverflow=off  RndMeth=Floor
  Data Type Conversion18 : DataTypeConversion  OutDataTypeStr=single  SaturateOnIntegerOverflow=off  RndMeth=Floor
  Data Type Conversion2 : DataTypeConversion  OutDataTypeStr=double  SaturateOnIntegerOverflow=off  RndMeth=Floor
  Data Type Conversion3 : DataTypeConversion  OutDataTypeStr=double  SaturateOnIntegerOverflow=off  RndMeth=Floor
  Zero-Order Hold{,1..3} (4 alike) : ZeroOrderHold  SampleTime=ts_afe
  modulator1 : Subsystem
  firing_gates : Outport
  wires:
  Zero-Order Hold2/1 -> C Caller/3
  Constant/1 -> Data Type Conversion16/1
  Data Type Conversion18/1 -> Zero-Order Hold/1
  enable/1 -> Data Type Conversion17/1
  Data Type Conversion16/1 -> Zero-Order Hold2/1
  Data Type Conversion17/1 -> Zero-Order Hold3/1
  Zero-Order Hold3/1 -> C Caller/4
  Data Type Conversion15/1 -> Zero-Order Hold1/1
  modulator1/1(cmd_gates) -> firing_gates/1
  Bus Selector1/1 -> Data Type Conversion18/1  "<ualpha_afe>"
  Bus Selector1/2 -> Data Type Conversion15/1  "<ubeta_afe>"
  Data Type Conversion3/1 -> modulator1/3(w)  "dw"
  Data Type Conversion2/1 -> modulator1/2(v)  "dv"
  Data Type Conversion1/1 -> modulator1/1(u)  "du"
  ab/1 -> Bus Selector1/1
  Zero-Order Hold/1 -> C Caller/1
  Zero-Order Hold1/1 -> C Caller/2
  C Caller/1 -> Bus Selector/1  "out"
  Bus Selector/1 -> Data Type Conversion1/1  "<da>"
  Bus Selector/2 -> Data Type Conversion2/1  "<db>"
  Bus Selector/3 -> Data Type Conversion3/1  "<dc>"

== system afe_dq_inv_psm/afe_dq_inv_psm_mod1/afe/switch_1 ==
  Diode : fl_lib/Electrical/Electrical Elements/Diode  Vf=Vgamma V  Ron=Ron Ohm  Goff=1e-8 1/Ohm  i_specify=off  i_priority=None  i=0 A  i_nominal_specify=off  i_nominal_value=1  i_nominal_unit=A  v_specify=off  v_priority=None  v=0 V  v_nominal_specify=off  v_nominal_value=1  v_nominal_unit=V
  Switch : fl_lib/Electrical/Electrical Elements/Switch  R_closed=Ron Ohm  G_open=1e-8 1/Ohm  Threshold=7.5  i_specify=off  i_priority=None  i=0 A  i_nominal_specify=off  i_nominal_value=1  i_nominal_unit=A  v_specify=off  v_priority=None  v=0 V  v_nominal_specify=off  v_nominal_value=1  v_nominal_unit=V
  snubber : fl_lib/Electrical/Electrical Elements/Capacitor  c=Csnubber F  r=Rsnubber Ohm  g=0 1/Ohm  i_specify=off  i_priority=None  i=0 A  i_nominal_specify=off  i_nominal_value=1  i_nominal_unit=A  v_specify=off  v_priority=None  v=0 V  v_nominal_specify=off  v_nominal_value=1  v_nominal_unit=V  vc_specify=off  vc_priority=High  vc=0 V  vc_nominal_specify=off  vc_nominal_value=1  vc_nominal_unit=V
  G : PMIOPort  Side=Left
  C : PMIOPort  Port=2  Side=Left
  E : PMIOPort  Port=3  Side=Right
  connections:
  Diode/LConn1 -- snubber/RConn1 -- E/RConn1 -- Switch/LConn1
  Switch/RConn1 -- G/RConn1
  Diode/RConn1 -- snubber/LConn1 -- C/RConn1 -- Switch/RConn2
